simulink model "ModeloNaoLinear"  (Simulink 7.1)
settings: Solver=ode45  StartTime=0.0  StopTime=10.0  RelTol=1e-3
settings Model: Creator=ALUNO  LastModifiedBy=ALUNO

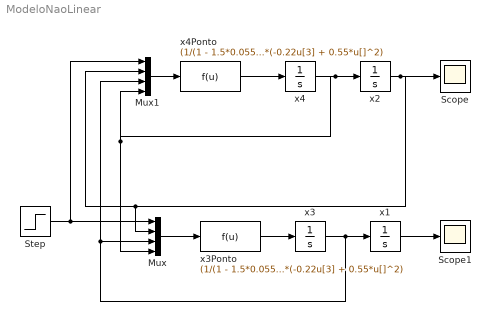
== system ModeloNaoLinear ==
  Mux : Mux
  Mux1 : Mux
  Scope : Scope
  Scope1 : Scope
  Step : Step  SampleTime=0
  x{1..4} (4 alike) : Integrator
  x3Ponto : Fcn  Expr=(1/(1 - 1.5*0.055*cos^2(u[2])))*(-0.22u[3] + 0.55*u[]^2)
  x4Ponto : Fcn  Expr=(1/(1 - 1.5*0.055*cos^2(u[2])))*(-0.22u[3] + 0.55*u[]^2)
  wires:
  Mux/1 -> x3Ponto/1
  x3Ponto/1 -> x3/1
  x3/1 -> x1/1, Mux/3, Mux1/3
  Step/1 -> Mux/1, Mux1/1
  x4Ponto/1 -> x4/1
  x4/1 -> x2/1, Mux/4, Mux1/4
  Mux1/1 -> x4Ponto/1
  x2/1 -> Mux/2, Mux1/2, Scope/1
  x1/1 -> Scope1/1
